simulink model "SingalFilter"  (R2022b)
settings: Solver=FixedStepAuto  StartTime=0.0  StopTime=10.0  RelTol=1e-3
settings Model: Creator=yuzehong  LastModifiedBy=yuzehong
settings OptimizationCC: DefaultParameterBehavior=Inlined  EnhancedBackFolding=on  PassReuseOutputArgsAs=Individual arguments  ZeroExternalMemoryAtStartup=off  ZeroInternalMemoryAtStartup=off  OptimizeBlockOrder=speed  DifferentSizesBufferReuse=on  OptimizationCustomize=off  EfficientTunableParamExpr=on
settings DebuggingCC: ParameterTunabilityLossMsg=error
settings SFSimCC: MATLABDynamicMemAlloc=off
settings RTWCC: Description=Embedded Coder  SystemTargetFile=ert.tlc  TemplateMakefile=ert_default_tmf
settings CodeAppCC: GenerateComments=off  IgnoreCustomStorageClasses=off  OperatorAnnotations=on  SimulinkDataObjDesc=on  SFDataObjDesc=on  SimulinkBlockComments=off
settings ERTTargetCC: TargetLangStandard=C99 (ISO)  GenerateSampleERTMain=on  InlinedParameterPlacement=NonHierarchical  ERTCustomFileTemplate=example_file_process.tlc

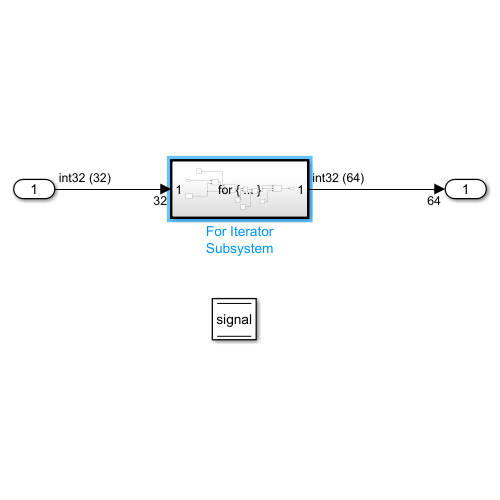
[thumbnail: Simulink's stored preview of the top-level diagram]
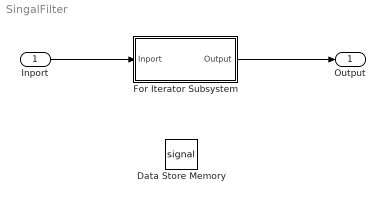
== system SingalFilter ==
  Inport : Inport  OutDataTypeStr=int32  PortDimensions=32
  Data Store Memory : DataStoreMemory  DataStoreName=signal  WriteAfterWriteMsg=warning  InitialValue=2  ShowAdditionalParam=off  OutDataTypeStr=int32  Dimensions=64
  For Iterator Subsystem : Subsystem  TreatAsAtomicUnit=on
  Output : Outport
  wires:
  For Iterator Subsystem/1(Output) -> Output/1
  Inport/1 -> For Iterator Subsystem/1(Inport)

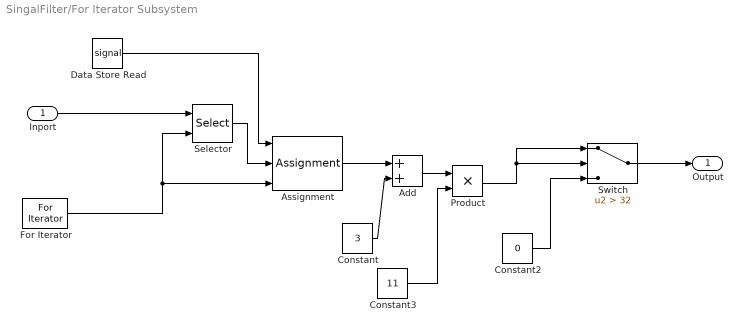
== system SingalFilter/For Iterator Subsystem ==
  Inport : Inport  PortDimensions=32
  Add : Sum  OutDataTypeStr=int32
  Assignment : Assignment  IndexMode=Zero-based  DiagnosticForDimensions=Warning  IndexOptions=Index vector (port)  Indices=1  OutputSizes=1
  Constant : Constant  Value=3  OutDataTypeStr=int32
  Constant2 : Constant  Value=0  OutDataTypeStr=int32
  Constant3 : Constant  Value=11  OutDataTypeStr=int32
  Data Store Read : DataStoreRead  DataStoreName=signal  IndexOptions=Index vector (dialog)  Indices=1  OutputSizes=1
  For Iterator : ForIterator  IterationLimit=32  IndexMode=Zero-based
  Product : Product  OutDataTypeStr=int32
  Selector : Selector  IndexMode=Zero-based  InputPortWidth=32  IndexOptions=Index vector (port)  Indices=[1 3]  OutputSizes=1
  Switch : Switch  Criteria=u2 > Threshold  Threshold=32  SaturateOnIntegerOverflow=off  InputSameDT=off
  Output : Outport
  wires:
  Constant2/1 -> Switch/3
  Switch/1 -> Output/1
  Inport/1 -> Selector/1
  For Iterator/1 -> Assignment/3, Selector/2
  Selector/1 -> Assignment/2
  Data Store Read/1 -> Assignment/1
  Assignment/1 -> Add/1
  Constant/1 -> Add/2
  Add/1 -> Product/1
  Constant3/1 -> Product/2
  Product/1 -> Switch/1, Switch/2
